simulink model "serial_test"  (R2013a)
settings: Solver=ode3  StartTime=0.0  StopTime=Inf  FixedStep=0.1  RelTol=1e-3
undefined symbols (not defined in the file): serial
libraries: instrumentlib x3
settings Model: Creator=nano  LastModifiedBy=nano

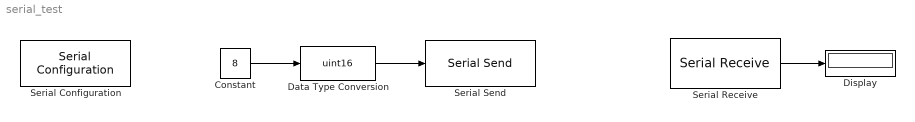
== system serial_test ==
  Constant : Constant  Value=8  SampleTime=0.1
  Data Type Conversion : DataTypeConversion  OutDataTypeStr=uint16
  Display : Display
  Serial Configuration : instrumentlib/Serial Configuration  Priority=-200000  ComPortMenu=COM6  ComPort=COM6  ObjConstructor=serial('COM6');  BaudRate=115200  DataBits=8  Parity=none  StopBits=1  FlowControl=none  Timeout=10  ByteOrder=LittleEndian
  Serial Receive : instrumentlib/Serial Receive  ComPortMenu=COM6  ComPort=COM6  ObjConstructor=serial('COM6');  Terminator=<none>  DataSize=[1 1]  DataType=uint16  EnableBlockingMode=on  ActionDataUnavailable=Output last received value  CustomValue=0  SampleTime=0.1
  Serial Send : instrumentlib/Serial Send  ComPortMenu=COM6  ComPort=COM6  ObjConstructor=serial('COM6');  Terminator=<none>  EnableBlockingMode=off
  wires:
  Serial Receive/1 -> Display/1
  Constant/1 -> Data Type Conversion/1
  Data Type Conversion/1 -> Serial Send/1
